simulink model "Position_Drift_Checking"  (R2015b)
settings: Solver=VariableStepAuto  StartTime=0.0  StopTime=100  RelTol=1e-3
values from neighbouring files (symbols this model uses):
  b = block.DialogPrm(1).Data    [controller_less.m]    (also in controller_more.m)
  m = 1    [Initiation.m]
undefined symbols (not defined in the file or in its folder): k, p
settings Model: Creator=TOSHIBA  LastModifiedBy=TOSHIBA

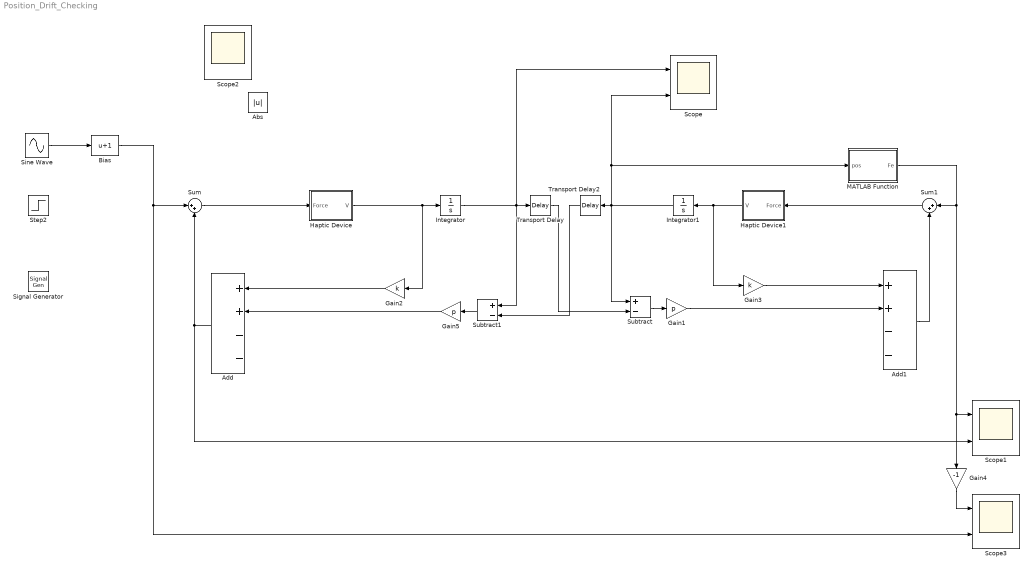
== system Position_Drift_Checking ==
  Abs : Abs
  Add : Sum  Inputs=++--
  Add1 : Sum  Inputs=++--
  Bias : Bias  Bias=1
  Gain1 : Gain  Gain=p
  Gain2 : Gain  Gain=k
  Gain3 : Gain  Gain=k
  Gain4 : Gain  Gain=-1
  Gain5 : Gain  Gain=p
  Haptic Device : Subsystem
  Haptic Device1 : Subsystem
  Integrator : Integrator
  Integrator1 : Integrator
  MATLAB Function : MATLAB Function  TreatAsAtomicUnit=on
  Scope{,1..3} (4 alike) : Scope  NumInputPorts=2
  Signal Generator : SignalGenerator  WaveForm=square  Amplitude=-1  Frequency=0.05*pi  Units=rad/sec
  Sine Wave : Sin  Amplitude=2  Frequency=pi/5  SampleTime=0
  Step2 : Step  Time=0  SampleTime=0
  Subtract : Sum  Inputs=+-
  Subtract1 : Sum  Inputs=+-
  Sum : Sum  Inputs=|++
  Sum1 : Sum  Inputs=|++
  Transport Delay : TransportDelay  DelayTime=t
  Transport Delay2 : TransportDelay  DelayTime=t
  wires:
  Haptic Device/1(V) -> Gain2/1, Integrator/1
  Haptic Device1/1(V) -> Gain3/1, Integrator1/1
  Integrator1/1 -> MATLAB Function/1(pos), Scope/2, Subtract/1, Transport Delay2/1
  Add1/1 -> Sum1/2
  Add/1 -> Scope1/2, Sum/2
  Subtract1/1 -> Gain5/1
  Transport Delay2/1 -> Subtract1/2
  Transport Delay/1 -> Subtract/2
  Subtract/1 -> Gain1/1
  MATLAB Function/1(Fe) -> Gain4/1, Scope1/1, Sum1/1
  Gain5/1 -> Add/2
  Gain1/1 -> Add1/2
  Integrator/1 -> Scope/1, Subtract1/1, Transport Delay/1
  Sum/1 -> Haptic Device/1(Force)
  Sum1/1 -> Haptic Device1/1(Force)
  Gain2/1 -> Add/1
  Gain3/1 -> Add1/1
  Sine Wave/1 -> Bias/1
  Gain4/1 -> Scope3/1
  Bias/1 -> Scope3/2, Sum/1

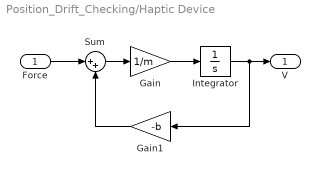
== system Position_Drift_Checking/Haptic Device ==
  Force : Inport
  Gain : Gain  Gain=1/m
  Gain1 : Gain  Gain=-b
  Integrator : Integrator
  Sum : Sum  Inputs=|++
  V : Outport
  wires:
  Gain/1 -> Integrator/1
  Sum/1 -> Gain/1
  Gain1/1 -> Sum/2
  Integrator/1 -> V/1, Gain1/1
  Force/1 -> Sum/1

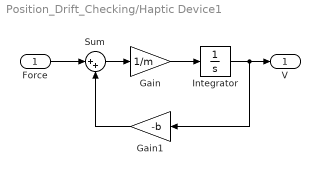
== system Position_Drift_Checking/Haptic Device1 ==
  Force : Inport
  Gain : Gain  Gain=1/m
  Gain1 : Gain  Gain=-b
  Integrator : Integrator
  Sum : Sum  Inputs=|++
  V : Outport
  wires:
  Force/1 -> Sum/1
  Integrator/1 -> Gain1/1, V/1
  Gain1/1 -> Sum/2
  Sum/1 -> Gain/1
  Gain/1 -> Integrator/1

== matlab function Position_Drift_Checking/MATLAB Function ==
  data: pos input; Fe output
function Fe = Envir(pos)
%#codegen
if pos>=0.05
    Fe=-(pos-0.05)*1000;
else
    Fe=0;
end
